simulink model "example_7_at_section"  (R2021a)
settings: Solver=VariableStepAuto  StartTime=0.0  StopTime=10.0  RelTol=1e-3
settings Model: Creator=YasserNet  LastModifiedBy=YasserNet

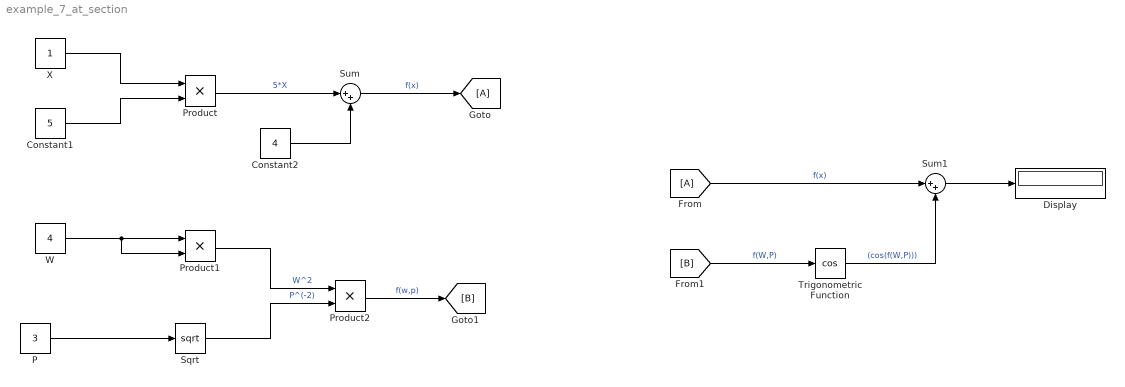
== system example_7_at_section ==
  Constant1 : Constant  Value=5
  Constant2 : Constant  Value=4
  Display : Display
  P : Constant  Value=3
  Product : Product
  Product1 : Product
  Product2 : Product
  Sqrt : Sqrt  SaturateOnIntegerOverflow=on
  Sum : Sum  Inputs=|++
  Sum1 : Sum  Inputs=|++
  Trigonometric Function : Trigonometry  Operator=cos
  W : Constant  Value=4
  X : Constant
  wires:
  Product/1 -> Sum/1  "5*X"
  X/1 -> Product/1
  Constant1/1 -> Product/2
  Constant2/1 -> Sum/2
  Sum/1 -> [A]  "f(x)"
  W/1 -> Product1/2, Product1/1
  P/1 -> Sqrt/1
  Product2/1 -> [B]  "f(w,p)"
  Product1/1 -> Product2/1  "W^2"
  Sqrt/1 -> Product2/2  "P^(-2)"
  [B] -> Trigonometric Function/1  "f(W,P)"
  Trigonometric Function/1 -> Sum1/2  "(cos(f(W,P)))"
  [A] -> Sum1/1  "f(x)"
  Sum1/1 -> Display/1
